simulink model "LAB3SIMULINK"  (R2017a)
settings: Solver=VariableStepAuto  StartTime=0.0  StopTime=0.8  RelTol=1e-3
values from neighbouring files (symbols this model uses):
  A_controlable = [0    1   0;                  0    0   1;                  -a0 -a1 -a2]    [PRELAB.m]
  A_ed = [-1*(R1+R2)/(R1*R2*C1)   1/(R2*C1)      -1/(R2*C1)     ;          0                 0              -1/(R3*C2)     ;        -1/(R2*C3)          1/(R2*C3)   -(R2+R3)/(R2*R3*C3)]    [PRELAB.m]
  A_LAT = linsys1.A    [PRELAB.m]
  A_observable = [-a2    1   0;                 -a1    0   1;                 -a0    0   0]    [PRELAB.m]
  B_controlable = [0;0;1]    [PRELAB.m]
  B_ed = [1/(R1*C1); 0; 0]    [PRELAB.m]
  B_LAT = linsys1.B    [PRELAB.m]
  B_observable = [b2; b1; b0]    [PRELAB.m]
  C_controlable = [b0,b1,b2]    [PRELAB.m]
  C_ed = [0 1 0]    [PRELAB.m]
  C_LAT = linsys1.C    [PRELAB.m]
  C_observable = [1,0,0]    [PRELAB.m]
  G0 = tf(b0,[1,a2,a1,a0])    [PRELAB.m]
undefined symbols (not defined in the file or in its folder): A_g0, B_g0, C_g0
settings Model: Creator=jacqu  LastModifiedBy=Gaby
settings SFSimCC: SimUseLocalCustomCode=on
settings RTWCC: RTWUseLocalCustomCode=on

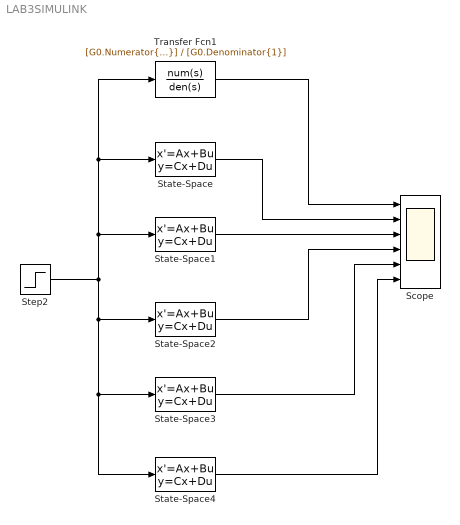
== system LAB3SIMULINK ==
  Scope : Scope  NumInputPorts=6
  State-Space : StateSpace  A=A_controlable  B=B_controlable  C=C_controlable  D=0  X0=0
  State-Space1 : StateSpace  A=A_observable  B=B_observable  C=C_observable  D=0  X0=0
  State-Space2 : StateSpace  A=A_ed  B=B_ed  C=C_ed  D=0  X0=0
  State-Space3 : StateSpace  A=A_g0  B=B_g0  C=C_g0  D=0  X0=0
  State-Space4 : StateSpace  A=A_LAT  B=B_LAT  C=C_LAT  D=0  X0=0
  Step2 : Step  Time=0.001  After=5  SampleTime=0
  Transfer Fcn1 : TransferFcn  Numerator=[G0.Numerator{1}]  Denominator=[G0.Denominator{1}]
  wires:
  Step2/1 -> Transfer Fcn1/1, State-Space/1, State-Space1/1, State-Space4/1, State-Space3/1, State-Space2/1
  Transfer Fcn1/1 -> Scope/1
  State-Space/1 -> Scope/2
  State-Space1/1 -> Scope/3
  State-Space2/1 -> Scope/4
  State-Space3/1 -> Scope/5
  State-Space4/1 -> Scope/6
